simulink model "gm_CustArch"  (R2020a)
settings: Solver=FixedStepDiscrete  StartTime=0.0  StopTime=7e4  RelTol=1e-3
libraries: simulink x85, hdlsllib x52, hdlmdlgenlib x2
(part 1 of 3)
settings Model: FPTRunName=FPA_Reference  Creator=BuccelliLab  LastModifiedBy=diflo
settings SolverCC: AutoInsertRateTranBlk=on  MinimalZcImpactIntegration=on
settings DataIOCC: LimitDataPoints=on  SaveOutput=off  SaveTime=off  ReturnWorkspaceOutputs=off
settings OptimizationCC: BlockReduction=off  ConditionallyExecuteInputs=off  DefaultParameterBehavior=Inlined  LifeSpan=inf
settings DebuggingCC: SignalRangeChecking=warning  ReadBeforeWriteMsg=DisableAll  WriteAfterWriteMsg=DisableAll  WriteAfterReadMsg=DisableAll  AlgebraicLoopMsg=error  ArtificialAlgebraicLoopMsg=none  InheritedTsInSrcMsg=none  MultiTaskDSMMsg=none  SingleTaskRateTransMsg=error  ParameterDowncastMsg=warning  ParameterOverflowMsg=warning  AllowSymbolicDim=off  StrictBusMsg=ErrorOnBusTreatedAsVector  SFUnexpectedBacktrackingDiag=warning  SFNoUnconditionalDefaultTransitionDiag=warning  SFExecutionAtInitializationDiag=none  ArithmeticOperatorsInVariantConditions=warning
settings HardwareCC: ProdBitPerPointer=32  ProdBitPerSizeT=32  ProdBitPerPtrDiffT=32  ProdLargestAtomicFloat=None  ProdIntDivRoundTo=Undefined  ProdEndianess=Unspecified  ProdWordSize=32  ProdHWDeviceType=ASIC/FPGA->ASIC/FPGA  TargetBitPerPointer=64  TargetBitPerSizeT=64  TargetBitPerPtrDiffT=64  TargetLongLongMode=on  TargetIntDivRoundTo=Zero  TargetEndianess=LittleEndian  TargetWordSize=64  TargetHWDeviceType=Custom Processor->MATLAB Host Computer  ProdEqTarget=off
settings ModelReferenceCC: UpdateModelReferenceTargets=IfOutOfDate
settings SFSimCC: SFSimEcho=off  SimUseLocalCustomCode=off  CustomCodeUndefinedFunction=UseInterfaceOnly
settings RTWCC: RTWUseLocalCustomCode=off
settings CodeAppCC: StateflowObjectComments=on
settings GRTTargetCC: TargetLangStandard=C89/C90 (ANSI)
settings ConfigComp: CovScope=ReferencedModels  CovMetricSettings=dw  CovHtmlReporting=on  CovSaveCumulativeToWorkspaceVar=on  CovSaveSingleToWorkspaceVar=on  CovExternalEMLEnable=off  CovSFcnEnable=off

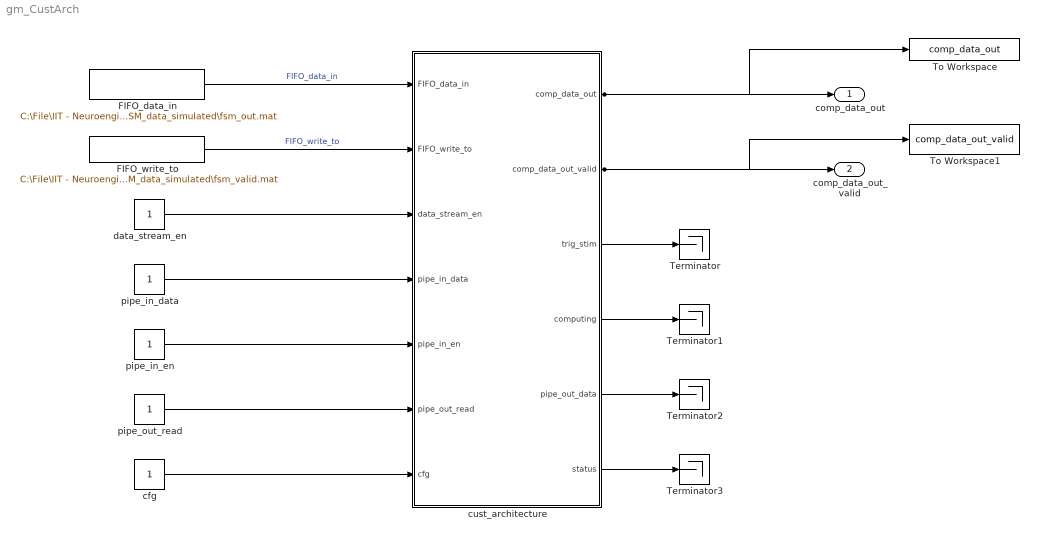
== system gm_CustArch ==
  FIFO_data_in : FromFile  FileName=C:\File\IIT - Neuroengineering\Progetto MathWorks\Data\Intan recordings\FSM_data_simulated\fsm_out.mat  OutDataTypeStr=uint16  SampleTime=1  ExtrapolationBeforeFirstDataPoint=Hold first value  InterpolationWithinTimeRange=Zero order hold  ExtrapolationAfterLastDataPoint=Hold last value
  FIFO_write_to : FromFile  FileName=C:\File\IIT - Neuroengineering\Progetto MathWorks\Data\Intan recordings\FSM_data_simulated\fsm_valid.mat  OutDataTypeStr=boolean  SampleTime=1
  Terminator{,1..3} (4 alike) : Terminator
  To Workspace : ToWorkspace  VariableName=comp_data_out  SaveFormat=Timeseries  SampleTime=-1
  To Workspace1 : ToWorkspace  VariableName=comp_data_out_valid  SaveFormat=Timeseries  SampleTime=-1
  cfg : Constant  OutDataTypeStr=uint16  SampleTime=-1
  cust_architecture : Subsystem
  data_stream_en : Constant  OutDataTypeStr=uint8  SampleTime=-1
  pipe_in_data : Constant  OutDataTypeStr=uint16  SampleTime=-1
  pipe_in_en : Constant  OutDataTypeStr=boolean  SampleTime=-1
  pipe_out_read : Constant  OutDataTypeStr=boolean  SampleTime=-1
  comp_data_out : Outport  VectorParamsAs1DForOutWhenUnconnected=off
  comp_data_out_valid : Outport  Port=2  VectorParamsAs1DForOutWhenUnconnected=off
  wires:
  cust_architecture/6(status) -> Terminator3/1
  cust_architecture/5(pipe_out_data) -> Terminator2/1
  cust_architecture/4(computing) -> Terminator1/1
  cust_architecture/3(trig_stim) -> Terminator/1
  cfg/1 -> cust_architecture/7(cfg)
  pipe_out_read/1 -> cust_architecture/6(pipe_out_read)
  pipe_in_en/1 -> cust_architecture/5(pipe_in_en)
  pipe_in_data/1 -> cust_architecture/4(pipe_in_data)
  data_stream_en/1 -> cust_architecture/3(data_stream_en)
  cust_architecture/2(comp_data_out_valid) -> comp_data_out_valid/1, To Workspace1/1
  cust_architecture/1(comp_data_out) -> comp_data_out/1, To Workspace/1
  FIFO_write_to/1 -> cust_architecture/2(FIFO_write_to)  "FIFO_write_to"
  FIFO_data_in/1 -> cust_architecture/1(FIFO_data_in)  "FIFO_data_in"

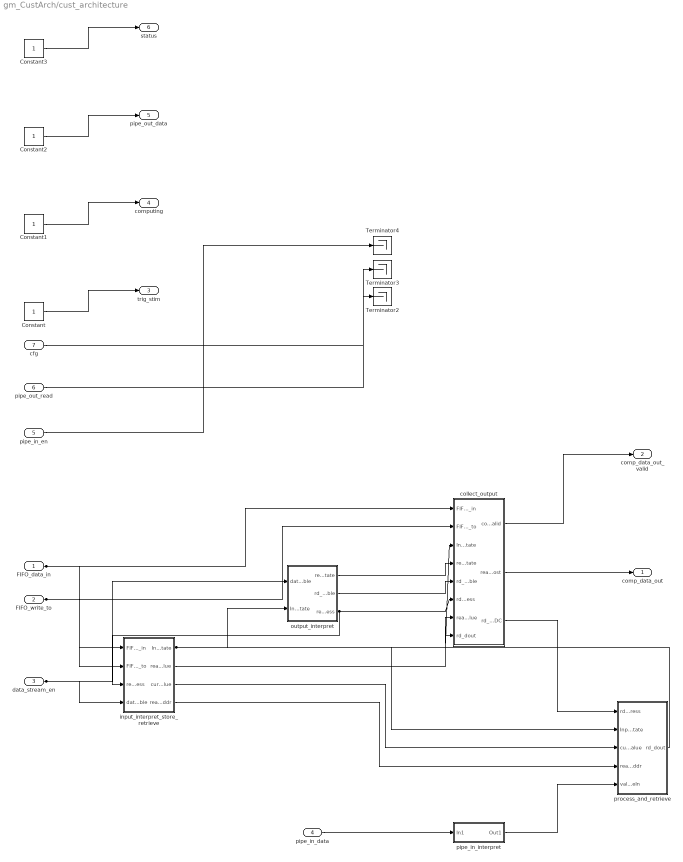
== system gm_CustArch/cust_architecture ==
  FIFO_data_in : Inport  OutDataTypeStr=uint16  PortDimensions=1  SampleTime=1
  FIFO_write_to : Inport  Port=2  OutDataTypeStr=boolean  PortDimensions=1  SampleTime=1
  data_stream_en : Inport  Port=3  OutDataTypeStr=uint8  PortDimensions=1  SampleTime=1
  pipe_in_data : Inport  Port=4  OutDataTypeStr=uint16  PortDimensions=1  SampleTime=1
  pipe_in_en : Inport  Port=5  OutDataTypeStr=boolean  PortDimensions=1  SampleTime=1
  pipe_out_read : Inport  Port=6  OutDataTypeStr=boolean  PortDimensions=1  SampleTime=1
  cfg : Inport  Port=7  OutDataTypeStr=uint16  PortDimensions=1  SampleTime=1
  Constant : Constant  OutDataTypeStr=uint8  SampleTime=1
  Constant1 : Constant  OutDataTypeStr=boolean  SampleTime=1
  Constant2 : Constant  OutDataTypeStr=uint16  SampleTime=1
  Constant3 : Constant  OutDataTypeStr=uint16  SampleTime=1
  Terminator2 : Terminator
  Terminator3 : Terminator
  Terminator4 : Terminator
  collect_output : Subsystem
  input_interpret_store_retrieve : Subsystem
  output_interpret : Subsystem
  pipe_in_interpret : Subsystem
  process_and_retrieve : Subsystem
  comp_data_out : Outport  VectorParamsAs1DForOutWhenUnconnected=off
  comp_data_out_valid : Outport  Port=2  OutDataTypeStr=boolean  VectorParamsAs1DForOutWhenUnconnected=off
  trig_stim : Outport  Port=3  VectorParamsAs1DForOutWhenUnconnected=off
  computing : Outport  Port=4  VectorParamsAs1DForOutWhenUnconnected=off
  pipe_out_data : Outport  Port=5  VectorParamsAs1DForOutWhenUnconnected=off
  status : Outport  Port=6  VectorParamsAs1DForOutWhenUnconnected=off
  wires:
  FIFO_data_in/1 -> input_interpret_store_retrieve/1(FIFO_data_in), collect_output/1(FIFO_data_in)
  FIFO_write_to/1 -> collect_output/2(FIFO_write_to), input_interpret_store_retrieve/2(FIFO_write_to)
  data_stream_en/1 -> output_interpret/1(data_stream_enable), input_interpret_store_retrieve/4(data_stream_enable)
  pipe_in_data/1 -> pipe_in_interpret/1(In1)
  pipe_in_en/1 -> Terminator4/1
  pipe_out_read/1 -> Terminator3/1
  cfg/1 -> Terminator2/1
  Constant/1 -> trig_stim/1
  Constant1/1 -> computing/1
  Constant2/1 -> pipe_out_data/1
  Constant3/1 -> status/1
  collect_output/1(comp_data_out_valid) -> comp_data_out_valid/1
  collect_output/2(read_from_storage_post) -> comp_data_out/1
  collect_output/3(rd_address_bit_set_AC_during_DC) -> process_and_retrieve/1(rd_address)
  input_interpret_store_retrieve/1(InputState) -> collect_output/3(InputState), output_interpret/2(InputState), process_and_retrieve/2(InputState)
  input_interpret_store_retrieve/2(read_from_storage_value) -> collect_output/7(read_from_storage_value)
  input_interpret_store_retrieve/3(current_value) -> process_and_retrieve/3(current_value)
  input_interpret_store_retrieve/4(read_from_processing_addr) -> process_and_retrieve/4(read_from_processing_addr)
  output_interpret/1(read_address == output_state) -> collect_output/4(read_address == output_state)
  output_interpret/2(rd_enable) -> collect_output/5(rd_enable)
  output_interpret/3(read_address) -> collect_output/6(rd_address), input_interpret_store_retrieve/3(read_address)
  pipe_in_interpret/1(Out1) -> process_and_retrieve/5(value_from_pipeIn)
  process_and_retrieve/1(rd_dout) -> collect_output/8(rd_dout)

== system gm_CustArch/cust_architecture/collect_output ==
  FIFO_data_in : Inport  OutDataTypeStr=uint16  PortDimensions=1  SampleTime=1
  FIFO_write_to : Inport  Port=2  OutDataTypeStr=boolean  PortDimensions=1  SampleTime=1
  InputState : Inport  Port=3  OutDataTypeStr=uint8  PortDimensions=1  SampleTime=1
  read_address == output_state : Inport  Port=4  OutDataTypeStr=uint8  PortDimensions=1  SampleTime=1
  rd_enable : Inport  Port=5  OutDataTypeStr=boolean  PortDimensions=1  SampleTime=1
  rd_address : Inport  Port=6  OutDataTypeStr=fixdt(0, 9, 0)  PortDimensions=1  SampleTime=1
  read_from_storage_value : Inport  Port=7  OutDataTypeStr=uint16  PortDimensions=1  SampleTime=1
  rd_dout : Inport  Port=8  OutDataTypeStr=uint16  PortDimensions=1  SampleTime=1
  AND : Logic  AllPortsSameDT=off  OutDataTypeStr=boolean  SampleTime=1
  Bit Set to get AC during DC : simulink/Logic and Bit Operations/Bit Set  iBit=0
      settings: SourceProductBaseCode=SL
  Compare To Constant : simulink/Logic and Bit Operations/Compare To Constant  relop=<  const="fi(0,0,8,0,\"hex\",\"06\")"  OutDataTypeStr=boolean
  Memory : UnitDelay  InitialCondition=double(0)  SampleTime=1
  Memory1 : UnitDelay  InitialCondition=double(0)  SampleTime=1
  Memory7 : UnitDelay  InitialCondition=double(0)  SampleTime=1
  Switch : Switch  Criteria=u2 > Threshold  Threshold=double(0)  OutDataTypeStr=uint16  SampleTime=1
  Switch2 : Switch  Criteria=u2 > Threshold  Threshold=double(0)  OutDataTypeStr=uint16  SampleTime=1
  get_data only when enabled : Subsystem
  output_state_DC : simulink/Logic and Bit Operations/Compare To Constant  relop=~=  const="fi(0,0,8,0,\"hex\",\"06\")"  OutDataTypeStr=boolean
  read_from_magic_and_timestamp : Subsystem
  comp_data_out_valid : Outport
  read_from_storage_post : Outport  Port=2
  rd_address_bit_set_AC_during_DC : Outport  Port=3
  wires:
  FIFO_data_in/1 -> read_from_magic_and_timestamp/2(FIFO_data_in)
  FIFO_write_to/1 -> read_from_magic_and_timestamp/3(FIFO_write_to)
  InputState/1 -> read_from_magic_and_timestamp/4(InputState)
  read_address == output_state/1 -> output_state_DC/1, Memory/1, read_from_magic_and_timestamp/1(read_address == output_state)
  rd_enable/1 -> Memory1/1
  rd_address/1 -> Bit Set to get AC during DC/1
  read_from_storage_value/1 -> Switch2/1
  rd_dout/1 -> Switch2/3
  AND/1 -> Switch/2
  Bit Set to get AC during DC/1 -> rd_address_bit_set_AC_during_DC/1
  Compare To Constant/1 -> AND/1
  Memory/1 -> Compare To Constant/1
  Memory1/1 -> AND/2, comp_data_out_valid/1, get_data only when enabled/Enable
  Memory7/1 -> Switch2/2
  Switch/1 -> get_data only when enabled/1(In1)
  Switch2/1 -> Switch/3
  get_data only when enabled/1(Out1) -> read_from_storage_post/1
  output_state_DC/1 -> Memory7/1
  read_from_magic_and_timestamp/1(read_from_Magic_TS) -> Switch/1

== system gm_CustArch/cust_architecture/input_interpret_store_retrieve ==
  FIFO_data_in : Inport  OutDataTypeStr=uint16  PortDimensions=1  SampleTime=1
  FIFO_write_to : Inport  Port=2  OutDataTypeStr=boolean  PortDimensions=1  SampleTime=1
  read_address : Inport  Port=3  OutDataTypeStr=fixdt(0, 9, 0)  PortDimensions=1  SampleTime=1
  data_stream_enable : Inport  Port=4  OutDataTypeStr=uint8  PortDimensions=1  SampleTime=1
  InputStateMachine : Subsystem
  Interpret_to_RAM_input : Subsystem
  store_and_retrieve_input : Subsystem
  InputState : Outport
  read_from_storage_value : Outport  Port=2
  current_value : Outport  Port=3
  read_from_processing_addr : Outport  Port=4
  wires:
  FIFO_data_in/1 -> InputStateMachine/1(FIFO_data_in), Interpret_to_RAM_input/1(FIFO_data_in)
  FIFO_write_to/1 -> InputStateMachine/2(FIFO_write_to), Interpret_to_RAM_input/2(FIFO_write_to)
  read_address/1 -> store_and_retrieve_input/1(read address)
  data_stream_enable/1 -> Interpret_to_RAM_input/4(data_stream_enable)
  InputStateMachine/1(InputState) -> InputState/1, Interpret_to_RAM_input/3(InputState)
  Interpret_to_RAM_input/1(device_output) -> InputStateMachine/3(channel_0_19)
  Interpret_to_RAM_input/2(inc_source_device) -> InputStateMachine/4(inc_source_device_MSB)
  Interpret_to_RAM_input/3(wr_din) -> store_and_retrieve_input/2(wr_din)
  Interpret_to_RAM_input/4(write address) -> store_and_retrieve_input/3(wr_address)
  Interpret_to_RAM_input/5(wr_en) -> store_and_retrieve_input/4(wr_en)
  store_and_retrieve_input/1(read_from_storage_value) -> read_from_storage_value/1
  store_and_retrieve_input/2(current value) -> current_value/1
  store_and_retrieve_input/3(read_from_porcessing_addr) -> read_from_processing_addr/1

== system gm_CustArch/cust_architecture/output_interpret ==
  data_stream_enable : Inport  OutDataTypeStr=uint8  PortDimensions=1  SampleTime=1
  InputState : Inport  Port=2  OutDataTypeStr=uint8  PortDimensions=1  SampleTime=1
  Interpret_to_RAM_output : Subsystem
  OutputStateMachine : Subsystem
  read_address == output_state : Outport
  rd_enable : Outport  Port=2
  read_address : Outport  Port=3
  wires:
  data_stream_enable/1 -> Interpret_to_RAM_output/2(data_stream_en)
  InputState/1 -> OutputStateMachine/1(input_state)
  Interpret_to_RAM_output/1(rd_enable) -> rd_enable/1
  Interpret_to_RAM_output/2(read address) -> read_address/1
  OutputStateMachine/1(OutputState) -> read_address == output_state/1, Interpret_to_RAM_output/1(read_address == output_state)

== system gm_CustArch/cust_architecture/pipe_in_interpret ==
  In1 : Inport  OutDataTypeStr=uint16  PortDimensions=1  SampleTime=1
  Bit Slice1 : hdlsllib/Logic and Bit Operations/Bit Slice  lidx=double(15)  ridx=double(8)
      settings: SourceProductBaseCode=SL
  Compare To Constant1 : simulink/Logic and Bit Operations/Compare To Constant  relop===  const="fi(0,0,8,0,\"hex\",\"02\")"  OutDataTypeStr=boolean
  Constant4 : Constant  Value=5  OutDataTypeStr=uint16  SampleTime=1
  Memory6 : UnitDelay  InitialCondition=double(0)  SampleTime=1
  Switch1 : Switch  Criteria=u2 > Threshold  Threshold=double(0)  OutDataTypeStr=uint16  SampleTime=1
  Out1 : Outport
  wires:
  In1/1 -> Switch1/1, Memory6/1
  Bit Slice1/1 -> Compare To Constant1/1
  Compare To Constant1/1 -> Switch1/2
  Constant4/1 -> Switch1/3
  Memory6/1 -> Bit Slice1/1
  Switch1/1 -> Out1/1

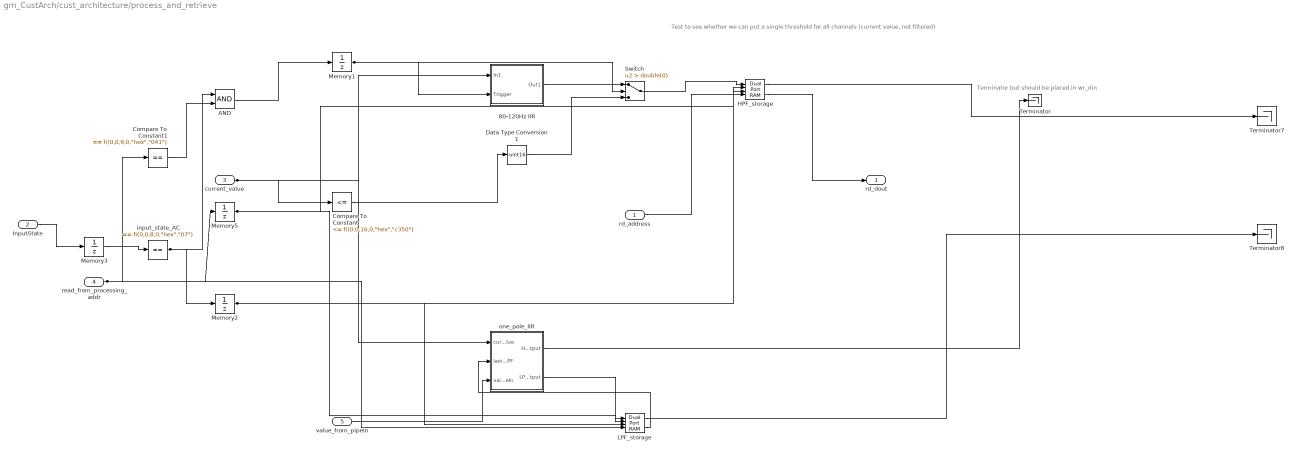
== system gm_CustArch/cust_architecture/process_and_retrieve ==
  note: Terminator but should be placed in wr_din
  note: Test to see whether we can put a single threshold for all channels (current value, not filtered)
  rd_address : Inport  OutDataTypeStr=fixdt(0, 9, 0)  PortDimensions=1  SampleTime=1
  InputState : Inport  Port=2  OutDataTypeStr=uint8  PortDimensions=1  SampleTime=1
  current_value : Inport  Port=3  OutDataTypeStr=uint16  PortDimensions=1  SampleTime=1
  read_from_processing_addr : Inport  Port=4  OutDataTypeStr=fixdt(0, 9, 0)  PortDimensions=1  SampleTime=1
  value_from_pipeIn : Inport  Port=5  OutDataTypeStr=uint16  PortDimensions=1  SampleTime=1
  80-120Hz IIR : Subsystem
  AND : Logic  AllPortsSameDT=off  OutDataTypeStr=boolean  SampleTime=1
  Compare To Constant : simulink/Logic and Bit Operations/Compare To Constant  relop=<=  const="fi(0,0,16,0,\"hex\",\"c350\")"  OutDataTypeStr=boolean
  Compare To Constant1 : simulink/Logic and Bit Operations/Compare To Constant  relop===  const="fi(0,0,9,0,\"hex\",\"041\")"  OutDataTypeStr=boolean
  Data Type Conversion1 : DataTypeConversion  OutDataTypeStr=uint16  SampleTime=1  SaturateOnIntegerOverflow=on
  HPF_storage : hdlsllib/HDL RAMs/Dual Port RAM  ram_size=9
      settings: SourceProductBaseCode=SL
  LPF_storage : hdlsllib/HDL RAMs/Dual Port RAM  ram_size=9
      settings: SourceProductBaseCode=SL
  Memory{1..3,5} (4 alike) : UnitDelay  InitialCondition=double(0)  SampleTime=1
  Switch : Switch  Criteria=u2 > Threshold  Threshold=double(0)  OutDataTypeStr=uint16  SampleTime=1
  Terminator : Terminator
  Terminator7 : Terminator
  Terminator8 : Terminator
  input_state_AC : simulink/Logic and Bit Operations/Compare To Constant  relop===  const="fi(0,0,8,0,\"hex\",\"07\")"  OutDataTypeStr=boolean
  one_pole_IIR : Subsystem
  rd_dout : Outport
  wires:
  rd_address/1 -> HPF_storage/4
  InputState/1 -> Memory3/1
  current_value/1 -> Compare To Constant/1, one_pole_IIR/1(current_value), 80-120Hz IIR/1(In1)
  read_from_processing_addr/1 -> Compare To Constant1/1, Memory5/1, LPF_storage/4
  value_from_pipeIn/1 -> one_pole_IIR/3(value_from_pipeIn)
  80-120Hz IIR/1(Out1) -> Switch/1
  AND/1 -> Memory1/1
  Compare To Constant/1 -> Data Type Conversion1/1
  Compare To Constant1/1 -> AND/2
  Data Type Conversion1/1 -> Switch/3
  HPF_storage/1 -> Terminator7/1
  HPF_storage/2 -> rd_dout/1
  LPF_storage/1 -> Terminator8/1
  LPF_storage/2 -> one_pole_IIR/2(last_LPF)
  Memory1/1 -> Switch/2, 80-120Hz IIR/2(Trigger)
  Memory2/1 -> HPF_storage/3, LPF_storage/3
  Memory3/1 -> input_state_AC/1
  Memory5/1 -> HPF_storage/2, LPF_storage/2
  Switch/1 -> HPF_storage/1
  input_state_AC/1 -> AND/1, Memory2/1
  one_pole_IIR/1(HPF_output) -> Terminator/1
  one_pole_IIR/2(LPF_output) -> LPF_storage/1

== system gm_CustArch/cust_architecture/collect_output/get_data only when enabled ==
  In1 : Inport  OutDataTypeStr=uint16  PortDimensions=1  SampleTime=1
  Enable : EnablePort  OutDataTypeStr=boolean
  Out1 : Outport  InitialOutput=0  VectorParamsAs1DForOutWhenUnconnected=off
  wires:
  In1/1 -> Out1/1

== system gm_CustArch/cust_architecture/collect_output/read_from_magic_and_timestamp ==
  read_address == output_state : Inport  OutDataTypeStr=uint8  PortDimensions=1  SampleTime=1
  FIFO_data_in : Inport  Port=2  OutDataTypeStr=uint16  PortDimensions=1  SampleTime=1
  FIFO_write_to : Inport  Port=3  OutDataTypeStr=boolean  PortDimensions=1  SampleTime=1
  InputState : Inport  Port=4  OutDataTypeStr=uint8  PortDimensions=1  SampleTime=1
  Terminator1 : Terminator
  getting address and enable for Magic and Timestamps : Subsystem
  input_RAM_for_MagicNumber_TimeStamps : hdlsllib/HDL RAMs/Dual Port RAM  ram_size=8
      settings: SourceProductBaseCode=SL
  read_from_Magic_TS : Outport
  wires:
  read_address == output_state/1 -> input_RAM_for_MagicNumber_TimeStamps/4
  FIFO_data_in/1 -> input_RAM_for_MagicNumber_TimeStamps/1
  FIFO_write_to/1 -> getting address and enable for Magic and Timestamps/2(FIFO_write_to)
  InputState/1 -> getting address and enable for Magic and Timestamps/1(InputState)
  getting address and enable for Magic and Timestamps/1(wr_address) -> input_RAM_for_MagicNumber_TimeStamps/2
  getting address and enable for Magic and Timestamps/2(wr_enable) -> input_RAM_for_MagicNumber_TimeStamps/3
  input_RAM_for_MagicNumber_TimeStamps/1 -> Terminator1/1
  input_RAM_for_MagicNumber_TimeStamps/2 -> read_from_Magic_TS/1

== system gm_CustArch/cust_architecture/input_interpret_store_retrieve/InputStateMachine ==
  FIFO_data_in : Inport  OutDataTypeStr=uint16  PortDimensions=1  SampleTime=1
  FIFO_write_to : Inport  Port=2  OutDataTypeStr=boolean  PortDimensions=1  SampleTime=1
  channel_0_19 : Inport  Port=3  OutDataTypeStr=uint8  PortDimensions=1  SampleTime=1
  inc_source_device_MSB : Inport  Port=4  OutDataTypeStr=boolean  PortDimensions=1  SampleTime=1
  InputStateMachine : Stateflow chart  TreatAsAtomicUnit=on
  InputState : Outport  VectorParamsAs1DForOutWhenUnconnected=off
  wires:
  FIFO_data_in/1 -> InputStateMachine/1(FIFO_data_in)
  FIFO_write_to/1 -> InputStateMachine/2(FIFO_write_to)
  channel_0_19/1 -> InputStateMachine/3(channel_0_19)
  inc_source_device_MSB/1 -> InputStateMachine/4(inc_source_device_MSB)
  InputStateMachine/1(InputState) -> InputState/1

== system gm_CustArch/cust_architecture/input_interpret_store_retrieve/Interpret_to_RAM_input ==
  FIFO_data_in : Inport  OutDataTypeStr=uint16  PortDimensions=1  SampleTime=1
  FIFO_write_to : Inport  Port=2  OutDataTypeStr=boolean  PortDimensions=1  SampleTime=1
  InputState : Inport  Port=3  OutDataTypeStr=uint8  PortDimensions=1  SampleTime=1
  data_stream_enable : Inport  Port=4  OutDataTypeStr=uint8  PortDimensions=1  SampleTime=1
  Input State to RAM address (to write) : Subsystem
  interpret data : Subsystem
  device_output : Outport
  inc_source_device : Outport  Port=2
  wr_din : Outport  Port=3
  write address : Outport  Port=4
  wr_en : Outport  Port=5
  wires:
  FIFO_data_in/1 -> Input State to RAM address (to write)/1(DataIn)
  FIFO_write_to/1 -> Input State to RAM address (to write)/6(write_to), interpret data/1(FIFO_write_to)
  InputState/1 -> Input State to RAM address (to write)/2(InputState), interpret data/2(InputState)
  data_stream_enable/1 -> interpret data/3(data_stream_enable)
  Input State to RAM address (to write)/1(wr_din) -> wr_din/1
  Input State to RAM address (to write)/2(wr_addr) -> write address/1
  Input State to RAM address (to write)/3(write_enable_6to15) -> wr_en/1
  interpret data/1(source_device) -> Input State to RAM address (to write)/4(source_device)
  interpret data/2(inc_source_device) -> inc_source_device/1
  interpret data/3(device_output) -> device_output/1
  interpret data/4(source_channel_0_159) -> Input State to RAM address (to write)/3(source_channel_0_159)
  interpret data/5(converter_cnt) -> Input State to RAM address (to write)/5(converter_cnt)

== system gm_CustArch/cust_architecture/input_interpret_store_retrieve/store_and_retrieve_input ==
  note: salvataggio dati su dual-ram, ogni dato ha un indirizzo associato
  note: così so l'indirizzo del dato
  read address : Inport  OutDataTypeStr=fixdt(0, 9, 0)  PortDimensions=1  SampleTime=1
  wr_din : Inport  Port=2  OutDataTypeStr=uint16  PortDimensions=1  SampleTime=1
  wr_address : Inport  Port=3  OutDataTypeStr=fixdt(0, 9, 0)  PortDimensions=1  SampleTime=1
  wr_en : Inport  Port=4  OutDataTypeStr=boolean  PortDimensions=1  SampleTime=1
  Memory4 : UnitDelay  InitialCondition=double(0)  SampleTime=1
  Terminator : Terminator
  Terminator6 : Terminator
  input_storage : hdlsllib/HDL RAMs/Dual Port RAM  ram_size=9
      settings: SourceProductBaseCode=SL
  input_storage_for_processing : hdlsllib/HDL RAMs/Dual Port RAM  ram_size=9
      settings: SourceProductBaseCode=SL
  read_from_storage_value : Outport
  current value : Outport  Port=2
  read_from_porcessing_addr : Outport  Port=3
  wires:
  read address/1 -> input_storage/4
  wr_din/1 -> input_storage/1, input_storage_for_processing/1
  wr_address/1 -> Memory4/1, input_storage/2, input_storage_for_processing/2
  wr_en/1 -> input_storage/3, input_storage_for_processing/3
  Memory4/1 -> read_from_porcessing_addr/1, input_storage_for_processing/4
  input_storage/1 -> Terminator/1
  input_storage/2 -> read_from_storage_value/1
  input_storage_for_processing/1 -> Terminator6/1
  input_storage_for_processing/2 -> current value/1

== system gm_CustArch/cust_architecture/output_interpret/Interpret_to_RAM_output ==
  read_address == output_state : Inport  OutDataTypeStr=uint8  PortDimensions=1  SampleTime=1
  data_stream_en : Inport  Port=2  OutDataTypeStr=uint8  PortDimensions=1  SampleTime=1
  Output State to RAM address (to read) : Subsystem
  "get enabled timings " : Subsystem
  rd_enable : Outport
  read address : Outport  Port=2
  wires:
  read_address == output_state/1 -> Output State to RAM address (to read)/3(OutputState), "get enabled timings "/1(output_state)
  data_stream_en/1 -> "get enabled timings "/2(data_stream_en)
  Output State to RAM address (to read)/1(rd_enable) -> rd_enable/1
  Output State to RAM address (to read)/2(rd_addr) -> read address/1
  "get enabled timings "/1(source_channel_en) -> Output State to RAM address (to read)/1(source_channel_en)
  "get enabled timings "/2(source_ch_0_159) -> Output State to RAM address (to read)/2(source_channel)
  "get enabled timings "/3(source_device_enabled) -> Output State to RAM address (to read)/4(source_device_en)
  "get enabled timings "/4(source_device) -> Output State to RAM address (to read)/5(source_device)
  "get enabled timings "/5(converter_cnt) -> Output State to RAM address (to read)/6(converter_cnt)

== system gm_CustArch/cust_architecture/output_interpret/OutputStateMachine ==
  input_state : Inport  OutDataTypeStr=uint8  PortDimensions=1  SampleTime=1
  OutputStateMachine : Stateflow chart  TreatAsAtomicUnit=on
  OutputState : Outport  VectorParamsAs1DForOutWhenUnconnected=off
  wires:
  input_state/1 -> OutputStateMachine/1(input_state)
  OutputStateMachine/1(OutputState) -> OutputState/1

== system gm_CustArch/cust_architecture/process_and_retrieve/80-120Hz IIR ==
  In1 : Inport  OutDataTypeStr=uint16  PortDimensions=1  SampleTime=1
  Trigger : Inport  Port=2  OutDataTypeStr=boolean  SampleTime=1
  Trigger_delay : Delay  DelayLength=double(1)  InitialCondition=1
  Trigger_delayed_inverted_and_Trigger : Logic  AllPortsSameDT=off  OutDataTypeStr=boolean  SampleTime=1
  controlss_temp : Subsystem
  not_Trigger_delayed : Logic  Operator=NOT  Inputs=1  AllPortsSameDT=off  OutDataTypeStr=boolean  SampleTime=1
  Out1 : Outport  InitialOutput=0
  wires:
  Trigger/1 -> Trigger_delayed_inverted_and_Trigger/2, Trigger_delay/1
  In1/1 -> controlss_temp/1(in0)
  controlss_temp/1(out0) -> Out1/1
  Trigger_delay/1 -> not_Trigger_delayed/1
  not_Trigger_delayed/1 -> Trigger_delayed_inverted_and_Trigger/1
  Trigger_delayed_inverted_and_Trigger/1 -> controlss_temp/2(Trigger_emulated)

== system gm_CustArch/cust_architecture/process_and_retrieve/one_pole_IIR ==
  current_value : Inport  OutDataTypeStr=uint16  PortDimensions=1  SampleTime=1
  last_LPF : Inport  Port=2  OutDataTypeStr=fixdt(1, 16, -5)  PortDimensions=1  SampleTime=1
  value_from_pipeIn : Inport  Port=3  OutDataTypeStr=uint16  PortDimensions=1  SampleTime=1
  Constant : Constant  Value=32768  OutDataTypeStr=uint16  SampleTime=1
  Constant1 : Constant  Value=32768  OutDataTypeStr=uint16  SampleTime=1
  Data Type Conversion1 : DataTypeConversion  OutDataTypeStr=int16  SampleTime=1  SaturateOnIntegerOverflow=on
  Filter1 : Subsystem
  Subtract1 : Sum  Inputs=+-  AccumDataTypeStr=fixdt(1, 17, 0)  OutDataTypeStr=int16  SampleTime=1
  Subtract2 : Sum  AccumDataTypeStr=fixdt(1, 18, 0)  OutDataTypeStr=uint16  SampleTime=1
  Terminator : Terminator
  HPF_output : Outport  VectorParamsAs1DForOutWhenUnconnected=off
  LPF_output : Outport  Port=2  VectorParamsAs1DForOutWhenUnconnected=off
  wires:
  current_value/1 -> Subtract1/1
  last_LPF/1 -> Filter1/2(Input1)
  value_from_pipeIn/1 -> Terminator/1
  Constant/1 -> Subtract1/2
  Constant1/1 -> Subtract2/2
  Data Type Conversion1/1 -> Subtract2/1
  Filter1/1(Output) -> Data Type Conversion1/1
  Filter1/2(Output1) -> LPF_output/1
  Subtract1/1 -> Filter1/1(Input)
  Subtract2/1 -> HPF_output/1

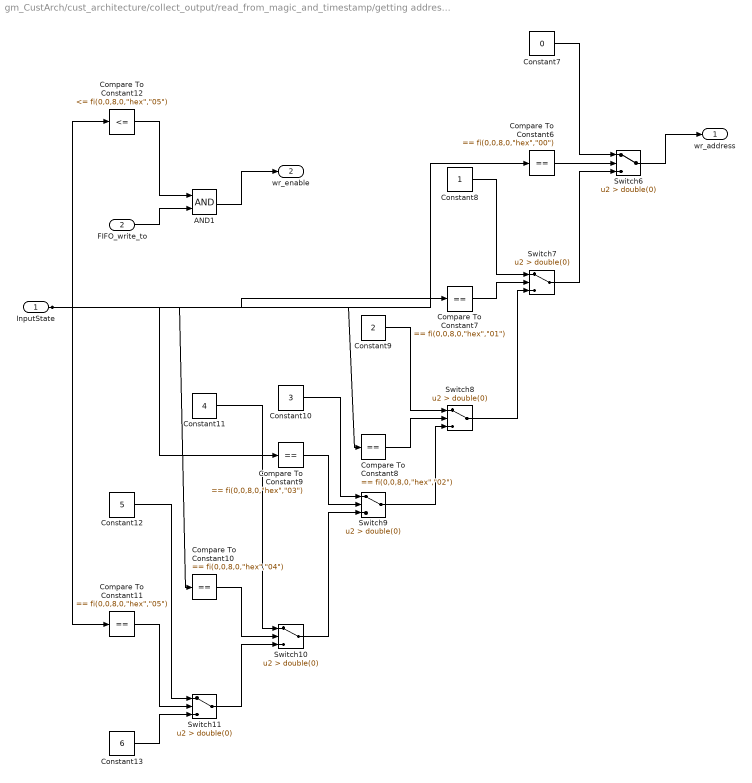
== system gm_CustArch/cust_architecture/collect_output/read_from_magic_and_timestamp/getting address and enable for Magic and Timestamps ==
  InputState : Inport  OutDataTypeStr=uint8  PortDimensions=1  SampleTime=1
  FIFO_write_to : Inport  Port=2  OutDataTypeStr=boolean  PortDimensions=1  SampleTime=1
  AND1 : Logic  AllPortsSameDT=off  OutDataTypeStr=boolean  SampleTime=1
  Compare To Constant10 : simulink/Logic and Bit Operations/Compare To Constant  relop===  const="fi(0,0,8,0,\"hex\",\"04\")"  OutDataTypeStr=boolean
  Compare To Constant11 : simulink/Logic and Bit Operations/Compare To Constant  relop===  const="fi(0,0,8,0,\"hex\",\"05\")"  OutDataTypeStr=boolean
  Compare To Constant12 : simulink/Logic and Bit Operations/Compare To Constant  relop=<=  const="fi(0,0,8,0,\"hex\",\"05\")"  OutDataTypeStr=boolean
  Compare To Constant6 : simulink/Logic and Bit Operations/Compare To Constant  relop===  const="fi(0,0,8,0,\"hex\",\"00\")"  OutDataTypeStr=boolean
  Compare To Constant7 : simulink/Logic and Bit Operations/Compare To Constant  relop===  const="fi(0,0,8,0,\"hex\",\"01\")"  OutDataTypeStr=boolean
  Compare To Constant8 : simulink/Logic and Bit Operations/Compare To Constant  relop===  const="fi(0,0,8,0,\"hex\",\"02\")"  OutDataTypeStr=boolean
  Compare To Constant9 : simulink/Logic and Bit Operations/Compare To Constant  relop===  const="fi(0,0,8,0,\"hex\",\"03\")"  OutDataTypeStr=boolean
  Constant10 : Constant  Value=3  OutDataTypeStr=uint8  SampleTime=1
  Constant11 : Constant  Value=4  OutDataTypeStr=uint8  SampleTime=1
  Constant12 : Constant  Value=5  OutDataTypeStr=uint8  SampleTime=1
  Constant13 : Constant  Value=6  OutDataTypeStr=uint8  SampleTime=1
  Constant7 : Constant  Value=0  OutDataTypeStr=uint8  SampleTime=1
  Constant8 : Constant  OutDataTypeStr=uint8  SampleTime=1
  Constant9 : Constant  Value=2  OutDataTypeStr=uint8  SampleTime=1
  Switch{6..11} (6 alike) : Switch  Criteria=u2 > Threshold  Threshold=double(0)  OutDataTypeStr=uint8  SampleTime=1
  wr_address : Outport  VectorParamsAs1DForOutWhenUnconnected=off
  wr_enable : Outport  Port=2  VectorParamsAs1DForOutWhenUnconnected=off
  wires:
  InputState/1 -> Compare To Constant9/1, Compare To Constant8/1, Compare To Constant7/1, Compare To Constant6/1, Compare To Constant12/1, Compare To Constant11/1, Compare To Constant10/1
  FIFO_write_to/1 -> AND1/2
  AND1/1 -> wr_enable/1
  Compare To Constant10/1 -> Switch10/2
  Compare To Constant11/1 -> Switch11/2
  Compare To Constant12/1 -> AND1/1
  Compare To Constant6/1 -> Switch6/2
  Compare To Constant7/1 -> Switch7/2
  Compare To Constant8/1 -> Switch8/2
  Compare To Constant9/1 -> Switch9/2
  Constant10/1 -> Switch9/1
  Constant11/1 -> Switch10/1
  Constant12/1 -> Switch11/1
  Constant13/1 -> Switch11/3
  Constant7/1 -> Switch6/1
  Constant8/1 -> Switch7/1
  Constant9/1 -> Switch8/1
  Switch10/1 -> Switch9/3
  Switch11/1 -> Switch10/3
  Switch6/1 -> wr_address/1
  Switch7/1 -> Switch6/3
  Switch8/1 -> Switch7/3
  Switch9/1 -> Switch8/3

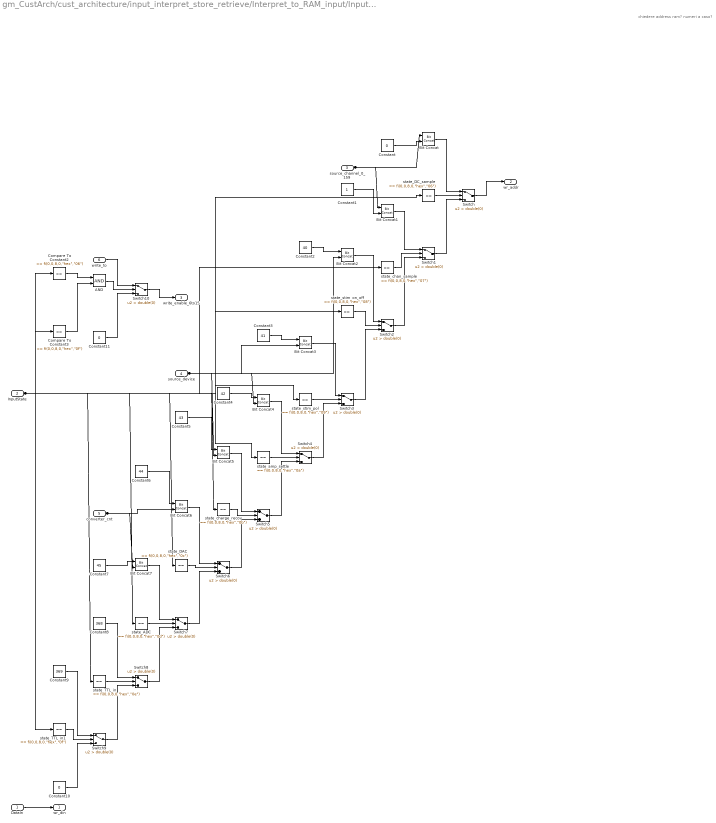
== system gm_CustArch/cust_architecture/input_interpret_store_retrieve/Interpret_to_RAM_input/Input State to RAM address (to write) ==
  note: chiedere address ram? numeri a caso?
  DataIn : Inport  OutDataTypeStr=uint16  PortDimensions=1  SampleTime=1
  InputState : Inport  Port=2  OutDataTypeStr=uint8  PortDimensions=1  SampleTime=1
  source_channel_0_159 : Inport  Port=3  OutDataTypeStr=uint8  PortDimensions=1  SampleTime=1
  source_device : Inport  Port=4  OutDataTypeStr=fixdt(0, 3, 0)  PortDimensions=1  SampleTime=1
  converter_cnt : Inport  Port=5  OutDataTypeStr=fixdt(0, 3, 0)  PortDimensions=1  SampleTime=1
  write_to : Inport  Port=6  OutDataTypeStr=boolean  PortDimensions=1  SampleTime=1
  AND : Logic  AllPortsSameDT=off  OutDataTypeStr=boolean  SampleTime=1
  Bit Concat{,1..7} (8 alike) : hdlsllib/Logic and Bit Operations/Bit Concat  numInputs=2
  Compare To Constant2 : simulink/Logic and Bit Operations/Compare To Constant  relop=>=  const="fi(0,0,8,0,\"hex\",\"06\")"  OutDataTypeStr=boolean
  Compare To Constant3 : simulink/Logic and Bit Operations/Compare To Constant  relop=<=  const="fi(0,0,8,0,\"hex\",\"0f\")"  OutDataTypeStr=boolean
  Constant : Constant  Value=0  OutDataTypeStr=boolean  SampleTime=1
  Constant1 : Constant  OutDataTypeStr=boolean  SampleTime=1
  Constant10 : Constant  Value=0  OutDataTypeStr=fixdt(0, 9, 1000)  SampleTime=1
  Constant11 : Constant  Value=0  OutDataTypeStr=boolean  SampleTime=1
  Constant2 : Constant  Value=40  OutDataTypeStr=fixdt(0, 6, 0)  SampleTime=1
  Constant3 : Constant  Value=41  OutDataTypeStr=fixdt(0, 6, 0)  SampleTime=1
  Constant4 : Constant  Value=42  OutDataTypeStr=fixdt(0, 6, 0)  SampleTime=1
  Constant5 : Constant  Value=43  OutDataTypeStr=fixdt(0, 6, 0)  SampleTime=1
  Constant6 : Constant  Value=44  OutDataTypeStr=fixdt(0, 6, 0)  SampleTime=1
  Constant7 : Constant  Value=45  OutDataTypeStr=fixdt(0, 6, 0)  SampleTime=1
  Constant8 : Constant  Value=368  OutDataTypeStr=fixdt(0, 9, 0)  SampleTime=1
  Constant9 : Constant  Value=369  OutDataTypeStr=fixdt(0, 9, 0)  SampleTime=1
  Switch{,1..9} (10 alike) : Switch  Criteria=u2 > Threshold  Threshold=double(0)  OutDataTypeStr=fixdt(0, 9, 0)  SampleTime=1
  Switch10 : Switch  Criteria=u2 > Threshold  Threshold=double(0)  OutDataTypeStr=boolean  SampleTime=1
  state_ADC : simulink/Logic and Bit Operations/Compare To Constant  relop===  const="fi(0,0,8,0,\"hex\",\"0d\")"  OutDataTypeStr=boolean
  state_DAC : simulink/Logic and Bit Operations/Compare To Constant  relop===  const="fi(0,0,8,0,\"hex\",\"0c\")"  OutDataTypeStr=boolean
  state_DC_sample : simulink/Logic and Bit Operations/Compare To Constant  relop===  const="fi(0,0,8,0,\"hex\",\"06\")"  OutDataTypeStr=boolean
  state_TTL_in : simulink/Logic and Bit Operations/Compare To Constant  relop===  const="fi(0,0,8,0,\"hex\",\"0e\")"  OutDataTypeStr=boolean
  state_TTL_in1 : simulink/Logic and Bit Operations/Compare To Constant  relop===  const="fi(0,0,8,0,\"hex\",\"0f\")"  OutDataTypeStr=boolean
  state_amp_settle : simulink/Logic and Bit Operations/Compare To Constant  relop===  const="fi(0,0,8,0,\"hex\",\"0a\")"  OutDataTypeStr=boolean
  state_chan_sample : simulink/Logic and Bit Operations/Compare To Constant  relop===  const="fi(0,0,8,0,\"hex\",\"07\")"  OutDataTypeStr=boolean
  state_charge_recov : simulink/Logic and Bit Operations/Compare To Constant  relop===  const="fi(0,0,8,0,\"hex\",\"0b\")"  OutDataTypeStr=boolean
  state_stim_on_off : simulink/Logic and Bit Operations/Compare To Constant  relop===  const="fi(0,0,8,0,\"hex\",\"08\")"  OutDataTypeStr=boolean
  state_stim_pol : simulink/Logic and Bit Operations/Compare To Constant  relop===  const="fi(0,0,8,0,\"hex\",\"09\")"  OutDataTypeStr=boolean
  wr_din : Outport  VectorParamsAs1DForOutWhenUnconnected=off
  wr_addr : Outport  Port=2  OutDataTypeStr=fixdt(0,9,0)  VectorParamsAs1DForOutWhenUnconnected=off
  write_enable_6to15 : Outport  Port=3  OutDataTypeStr=boolean  VectorParamsAs1DForOutWhenUnconnected=off
  wires:
  DataIn/1 -> wr_din/1
  InputState/1 -> state_stim_pol/1, state_stim_on_off/1, state_charge_recov/1, state_chan_sample/1, state_amp_settle/1, state_TTL_in1/1, state_TTL_in/1, state_DC_sample/1, state_DAC/1, state_ADC/1, Compare To Constant3/1, Compare To Constant2/1
  source_channel_0_159/1 -> Bit Concat1/1, Bit Concat/1
  source_device/1 -> Bit Concat5/2, Bit Concat4/2, Bit Concat3/2, Bit Concat2/2
  converter_cnt/1 -> Bit Concat7/2, Bit Concat6/2
  write_to/1 -> Switch10/1
  AND/1 -> Switch10/2
  Bit Concat/1 -> Switch/1
  Bit Concat1/1 -> Switch1/1
  Bit Concat2/1 -> Switch2/1
  Bit Concat3/1 -> Switch3/1
  Bit Concat4/1 -> Switch4/1
  Bit Concat5/1 -> Switch5/1
  Bit Concat6/1 -> Switch6/1
  Bit Concat7/1 -> Switch7/1
  Compare To Constant2/1 -> AND/1
  Compare To Constant3/1 -> AND/2
  Constant/1 -> Bit Concat/2
  Constant1/1 -> Bit Concat1/2
  Constant10/1 -> Switch9/3
  Constant11/1 -> Switch10/3
  Constant2/1 -> Bit Concat2/1
  Constant3/1 -> Bit Concat3/1
  Constant4/1 -> Bit Concat4/1
  Constant5/1 -> Bit Concat5/1
  Constant6/1 -> Bit Concat6/1
  Constant7/1 -> Bit Concat7/1
  Constant8/1 -> Switch8/1
  Constant9/1 -> Switch9/1
  Switch/1 -> wr_addr/1
  Switch1/1 -> Switch/3
  Switch10/1 -> write_enable_6to15/1
  Switch2/1 -> Switch1/3
  Switch3/1 -> Switch2/3
  Switch4/1 -> Switch3/3
  Switch5/1 -> Switch4/3
  Switch6/1 -> Switch5/3
  Switch7/1 -> Switch6/3
  Switch8/1 -> Switch7/3
  Switch9/1 -> Switch8/3
  state_ADC/1 -> Switch7/2
  state_DAC/1 -> Switch6/2
  state_DC_sample/1 -> Switch/2
  state_TTL_in/1 -> Switch8/2
  state_TTL_in1/1 -> Switch9/2
  state_amp_settle/1 -> Switch4/2
  state_chan_sample/1 -> Switch1/2
  state_charge_recov/1 -> Switch5/2
  state_stim_on_off/1 -> Switch2/2
  state_stim_pol/1 -> Switch3/2

== system gm_CustArch/cust_architecture/input_interpret_store_retrieve/Interpret_to_RAM_input/interpret data ==
  note: check ADC/DAC states
  note: count number of ADC/DAC states
  FIFO_write_to : Inport  OutDataTypeStr=boolean  PortDimensions=1  SampleTime=1
  InputState : Inport  Port=2  OutDataTypeStr=uint8  PortDimensions=1  SampleTime=1
  data_stream_enable : Inport  Port=3  OutDataTypeStr=uint8  PortDimensions=1  SampleTime=1
  Bit Slice : hdlsllib/Logic and Bit Operations/Bit Slice  lidx=double(2)  ridx=double(0)
      settings: SourceProductBaseCode=SL
  Bit Slice1 : hdlsllib/Logic and Bit Operations/Bit Slice  lidx=double(2)  ridx=double(0)
      settings: SourceProductBaseCode=SL
  HDL Counter : hdlsllib/Sources/HDL Counter  CountType=Count limited  CountInit=double(0)  CountStep=double(1)  CountMax=double(7)  CountFromType=Initial value  CountFrom=double(0)  CountResetPort=off  CountLoadPort=off  CountEnbPort=on  CountDirPort=off  CountDataType=Unsigned  CountWordLen=8  CountFracLen=0  CountSampTime=1
  "condition to count DAC or ADC " : Subsystem
  get_sources : Subsystem
  source_device : Outport  VectorParamsAs1DForOutWhenUnconnected=off
  inc_source_device : Outport  Port=2  VectorParamsAs1DForOutWhenUnconnected=off
  device_output : Outport  Port=3  VectorParamsAs1DForOutWhenUnconnected=off
  source_channel_0_159 : Outport  Port=4  VectorParamsAs1DForOutWhenUnconnected=off
  converter_cnt : Outport  Port=5  VectorParamsAs1DForOutWhenUnconnected=off
  wires:
  FIFO_write_to/1 -> "condition to count DAC or ADC "/1(fifo_write_to), get_sources/1(FIFO_write_to)
  InputState/1 -> "condition to count DAC or ADC "/2(input_state), get_sources/2(InputState)
  data_stream_enable/1 -> get_sources/3(data_stream_enable)
  Bit Slice/1 -> converter_cnt/1
  Bit Slice1/1 -> source_device/1
  HDL Counter/1 -> Bit Slice/1
  "condition to count DAC or ADC "/1(Out1) -> HDL Counter/1
  get_sources/1(source_device) -> Bit Slice1/1
  get_sources/2(dev_out_channel_0_19) -> device_output/1
  get_sources/3(source_channel) -> source_channel_0_159/1
  get_sources/4(bitmasked==0) -> inc_source_device/1

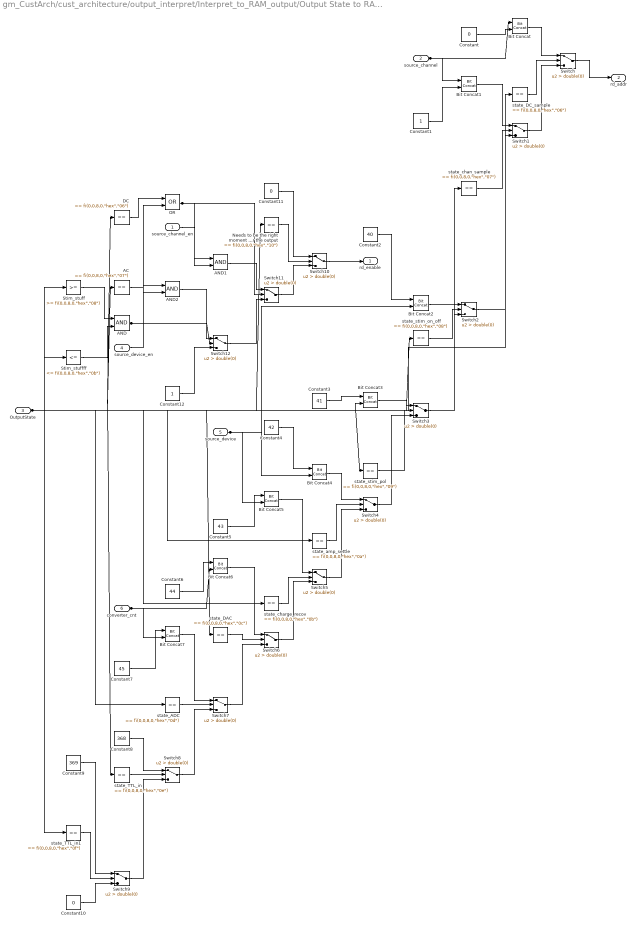
== system gm_CustArch/cust_architecture/output_interpret/Interpret_to_RAM_output/Output State to RAM address (to read) ==
  source_channel_en : Inport  OutDataTypeStr=boolean  PortDimensions=1  SampleTime=1
  source_channel : Inport  Port=2  OutDataTypeStr=uint8  PortDimensions=1  SampleTime=1
  OutputState : Inport  Port=3  OutDataTypeStr=uint8  PortDimensions=1  SampleTime=1
  source_device_en : Inport  Port=4  OutDataTypeStr=fixdt(0, 1, 0)  PortDimensions=1  SampleTime=1
  source_device : Inport  Port=5  OutDataTypeStr=fixdt(0, 3, 0)  PortDimensions=1  SampleTime=1
  converter_cnt : Inport  Port=6  OutDataTypeStr=fixdt(0, 3, 0)  PortDimensions=1  SampleTime=1
  AC : simulink/Logic and Bit Operations/Compare To Constant  relop===  const="fi(0,0,8,0,\"hex\",\"07\")"  OutDataTypeStr=boolean
  AND : Logic  AllPortsSameDT=off  OutDataTypeStr=boolean  SampleTime=1
  AND1 : Logic  AllPortsSameDT=off  OutDataTypeStr=boolean  SampleTime=1
  AND2 : Logic  AllPortsSameDT=off  OutDataTypeStr=boolean  SampleTime=1
  Bit Concat{,1..7} (8 alike) : hdlsllib/Logic and Bit Operations/Bit Concat  numInputs=2
  Constant : Constant  Value=0  OutDataTypeStr=boolean  SampleTime=1
  Constant1 : Constant  OutDataTypeStr=boolean  SampleTime=1
  Constant10 : Constant  Value=0  OutDataTypeStr=fixdt(0, 9, 1000)  SampleTime=1
  Constant11 : Constant  Value=0  OutDataTypeStr=boolean  SampleTime=1
  Constant12 : Constant  OutDataTypeStr=boolean  SampleTime=1
  Constant2 : Constant  Value=40  OutDataTypeStr=fixdt(0, 6, 0)  SampleTime=1
  Constant3 : Constant  Value=41  OutDataTypeStr=fixdt(0, 6, 0)  SampleTime=1
  Constant4 : Constant  Value=42  OutDataTypeStr=fixdt(0, 6, 0)  SampleTime=1
  Constant5 : Constant  Value=43  OutDataTypeStr=fixdt(0, 6, 0)  SampleTime=1
  Constant6 : Constant  Value=44  OutDataTypeStr=fixdt(0, 6, 0)  SampleTime=1
  Constant7 : Constant  Value=45  OutDataTypeStr=fixdt(0, 6, 0)  SampleTime=1
  Constant8 : Constant  Value=368  OutDataTypeStr=fixdt(0, 9, 0)  SampleTime=1
  Constant9 : Constant  Value=369  OutDataTypeStr=fixdt(0, 9, 0)  SampleTime=1
  DC : simulink/Logic and Bit Operations/Compare To Constant  relop===  const="fi(0,0,8,0,\"hex\",\"06\")"  OutDataTypeStr=boolean
  Needs to be the right moment for the output : simulink/Logic and Bit Operations/Compare To Constant  relop===  const="fi(0,0,8,0,\"hex\",\"10\")"  OutDataTypeStr=boolean
  OR : Logic  Operator=OR  AllPortsSameDT=off  OutDataTypeStr=boolean  SampleTime=1
  Stim_stuff : simulink/Logic and Bit Operations/Compare To Constant  relop=>=  const="fi(0,0,8,0,\"hex\",\"08\")"  OutDataTypeStr=boolean
  Stim_stuffff : simulink/Logic and Bit Operations/Compare To Constant  relop=<=  const="fi(0,0,8,0,\"hex\",\"0b\")"  OutDataTypeStr=boolean
  Switch{,1..9} (10 alike) : Switch  Criteria=u2 > Threshold  Threshold=double(0)  OutDataTypeStr=fixdt(0, 9, 0)  SampleTime=1
  Switch10 : Switch  Criteria=u2 > Threshold  Threshold=double(0)  OutDataTypeStr=boolean  SampleTime=1
  Switch11 : Switch  Criteria=u2 > Threshold  Threshold=double(0)  OutDataTypeStr=boolean  SampleTime=1
  Switch12 : Switch  Criteria=u2 > Threshold  Threshold=double(0)  OutDataTypeStr=boolean  SampleTime=1
  state_ADC : simulink/Logic and Bit Operations/Compare To Constant  relop===  const="fi(0,0,8,0,\"hex\",\"0d\")"  OutDataTypeStr=boolean
  state_DAC : simulink/Logic and Bit Operations/Compare To Constant  relop===  const="fi(0,0,8,0,\"hex\",\"0c\")"  OutDataTypeStr=boolean
  state_DC_sample : simulink/Logic and Bit Operations/Compare To Constant  relop===  const="fi(0,0,8,0,\"hex\",\"06\")"  OutDataTypeStr=boolean
  state_TTL_in : simulink/Logic and Bit Operations/Compare To Constant  relop===  const="fi(0,0,8,0,\"hex\",\"0e\")"  OutDataTypeStr=boolean
  state_TTL_in1 : simulink/Logic and Bit Operations/Compare To Constant  relop===  const="fi(0,0,8,0,\"hex\",\"0f\")"  OutDataTypeStr=boolean
  state_amp_settle : simulink/Logic and Bit Operations/Compare To Constant  relop===  const="fi(0,0,8,0,\"hex\",\"0a\")"  OutDataTypeStr=boolean
  state_chan_sample : simulink/Logic and Bit Operations/Compare To Constant  relop===  const="fi(0,0,8,0,\"hex\",\"07\")"  OutDataTypeStr=boolean
  state_charge_recov : simulink/Logic and Bit Operations/Compare To Constant  relop===  const="fi(0,0,8,0,\"hex\",\"0b\")"  OutDataTypeStr=boolean
  state_stim_on_off : simulink/Logic and Bit Operations/Compare To Constant  relop===  const="fi(0,0,8,0,\"hex\",\"08\")"  OutDataTypeStr=boolean
  state_stim_pol : simulink/Logic and Bit Operations/Compare To Constant  relop===  const="fi(0,0,8,0,\"hex\",\"09\")"  OutDataTypeStr=boolean
  rd_enable : Outport  VectorParamsAs1DForOutWhenUnconnected=off
  rd_addr : Outport  Port=2  OutDataTypeStr=fixdt(0,9,0)  VectorParamsAs1DForOutWhenUnconnected=off
  wires:
  source_channel_en/1 -> AND1/2
  source_channel/1 -> Bit Concat1/1, Bit Concat/1
  OutputState/1 -> state_stim_pol/1, state_stim_on_off/1, state_charge_recov/1, state_chan_sample/1, state_amp_settle/1, state_TTL_in1/1, state_TTL_in/1, state_DC_sample/1, state_DAC/1, state_ADC/1, Stim_stuffff/1, Stim_stuff/1, Needs to be the right moment for the output/1, DC/1, AC/1
  source_device_en/1 -> AND2/2
  source_device/1 -> Bit Concat5/2, Bit Concat4/2, Bit Concat3/2, Bit Concat2/2
  converter_cnt/1 -> Bit Concat7/2, Bit Concat6/2
  AC/1 -> OR/2
  AND/1 -> Switch12/2, AND2/1
  AND1/1 -> Switch11/1
  AND2/1 -> Switch12/1
  Bit Concat/1 -> Switch/1
  Bit Concat1/1 -> Switch1/1
  Bit Concat2/1 -> Switch2/1
  Bit Concat3/1 -> Switch3/1
  Bit Concat4/1 -> Switch4/1
  Bit Concat5/1 -> Switch5/1
  Bit Concat6/1 -> Switch6/1
  Bit Concat7/1 -> Switch7/1
  Constant/1 -> Bit Concat/2
  Constant1/1 -> Bit Concat1/2
  Constant10/1 -> Switch9/3
  Constant11/1 -> Switch10/1
  Constant12/1 -> Switch12/3
  Constant2/1 -> Bit Concat2/1
  Constant3/1 -> Bit Concat3/1
  Constant4/1 -> Bit Concat4/1
  Constant5/1 -> Bit Concat5/1
  Constant6/1 -> Bit Concat6/1
  Constant7/1 -> Bit Concat7/1
  Constant8/1 -> Switch8/1
  Constant9/1 -> Switch9/1
  DC/1 -> OR/1
  Needs to be the right moment for the output/1 -> Switch10/2
  OR/1 -> Switch11/2, AND1/1
  Stim_stuff/1 -> AND/1
  Stim_stuffff/1 -> AND/2
  Switch/1 -> rd_addr/1
  Switch1/1 -> Switch/3
  Switch10/1 -> rd_enable/1
  Switch11/1 -> Switch10/3
  Switch12/1 -> Switch11/3
  Switch2/1 -> Switch1/3
  Switch3/1 -> Switch2/3
  Switch4/1 -> Switch3/3
  Switch5/1 -> Switch4/3
  Switch6/1 -> Switch5/3
  Switch7/1 -> Switch6/3
  Switch8/1 -> Switch7/3
  Switch9/1 -> Switch8/3
  state_ADC/1 -> Switch7/2
  state_DAC/1 -> Switch6/2
  state_DC_sample/1 -> Switch/2
  state_TTL_in/1 -> Switch8/2
  state_TTL_in1/1 -> Switch9/2
  state_amp_settle/1 -> Switch4/2
  state_chan_sample/1 -> Switch1/2
  state_charge_recov/1 -> Switch5/2
  state_stim_on_off/1 -> Switch2/2
  state_stim_pol/1 -> Switch3/2

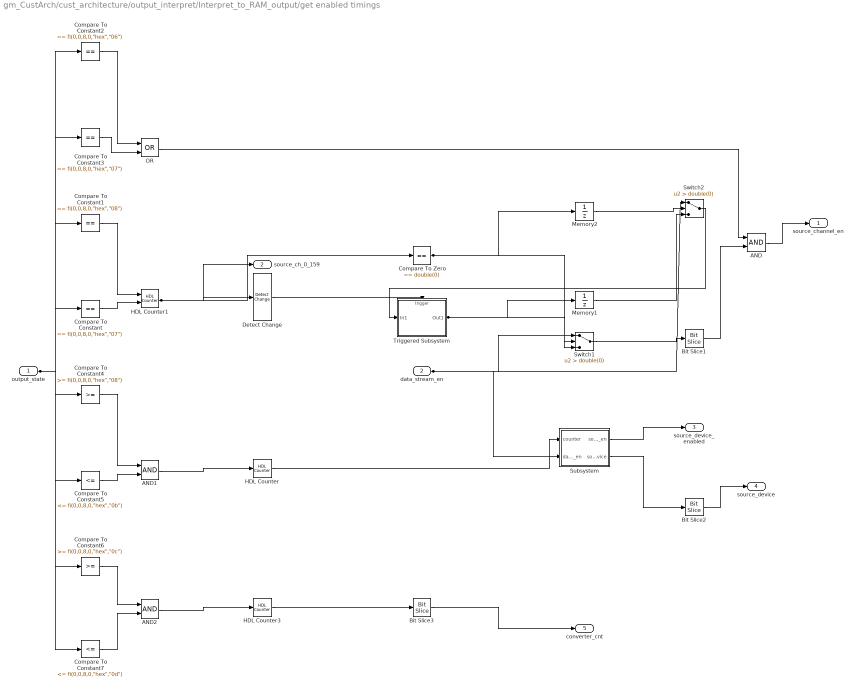
== system gm_CustArch/cust_architecture/output_interpret/Interpret_to_RAM_output/get enabled timings  ==
  output_state : Inport  OutDataTypeStr=uint8  PortDimensions=1  SampleTime=1
  data_stream_en : Inport  Port=2  OutDataTypeStr=uint8  PortDimensions=1  SampleTime=1
  AND : Logic  AllPortsSameDT=off  OutDataTypeStr=boolean  SampleTime=1
  AND1 : Logic  AllPortsSameDT=off  OutDataTypeStr=boolean  SampleTime=1
  AND2 : Logic  AllPortsSameDT=off  OutDataTypeStr=boolean  SampleTime=1
  Bit Slice1 : hdlsllib/Logic and Bit Operations/Bit Slice  lidx=double(0)  ridx=double(0)
      settings: SourceProductBaseCode=SL
  Bit Slice2 : hdlsllib/Logic and Bit Operations/Bit Slice  lidx=double(2)  ridx=double(0)
      settings: SourceProductBaseCode=SL
  Bit Slice3 : hdlsllib/Logic and Bit Operations/Bit Slice  lidx=double(2)  ridx=double(0)
      settings: SourceProductBaseCode=SL
  Compare To Constant : simulink/Logic and Bit Operations/Compare To Constant  relop===  const="fi(0,0,8,0,\"hex\",\"07\")"  OutDataTypeStr=boolean
  Compare To Constant1 : simulink/Logic and Bit Operations/Compare To Constant  relop===  const="fi(0,0,8,0,\"hex\",\"08\")"  OutDataTypeStr=boolean
  Compare To Constant2 : simulink/Logic and Bit Operations/Compare To Constant  relop===  const="fi(0,0,8,0,\"hex\",\"06\")"  OutDataTypeStr=boolean
  Compare To Constant3 : simulink/Logic and Bit Operations/Compare To Constant  relop===  const="fi(0,0,8,0,\"hex\",\"07\")"  OutDataTypeStr=boolean
  Compare To Constant4 : simulink/Logic and Bit Operations/Compare To Constant  relop=>=  const="fi(0,0,8,0,\"hex\",\"08\")"  OutDataTypeStr=boolean
  Compare To Constant5 : simulink/Logic and Bit Operations/Compare To Constant  relop=<=  const="fi(0,0,8,0,\"hex\",\"0b\")"  OutDataTypeStr=boolean
  Compare To Constant6 : simulink/Logic and Bit Operations/Compare To Constant  relop=>=  const="fi(0,0,8,0,\"hex\",\"0c\")"  OutDataTypeStr=boolean
  Compare To Constant7 : simulink/Logic and Bit Operations/Compare To Constant  relop=<=  const="fi(0,0,8,0,\"hex\",\"0d\")"  OutDataTypeStr=boolean
  Compare To Zero : simulink/Logic and Bit Operations/Compare To Constant  relop===  const=double(0)  OutDataTypeStr=boolean
  Detect Change : simulink/Logic and Bit Operations/Detect Change  vinit=0  OutDataTypeStr=boolean
  HDL Counter : hdlsllib/Sources/HDL Counter  CountType=Count limited  CountInit=double(0)  CountStep=double(1)  CountMax=double(7)  CountFromType=Initial value  CountFrom=double(0)  CountResetPort=off  CountLoadPort=off  CountEnbPort=on  CountDirPort=off  CountDataType=Unsigned  CountWordLen=8  CountFracLen=0  CountSampTime=1
  HDL Counter1 : hdlsllib/Sources/HDL Counter  CountType=Count limited  CountInit=double(0)  CountStep=double(1)  CountMax=double(159)  CountFromType=Initial value  CountFrom=double(0)  CountResetPort=on  CountLoadPort=off  CountEnbPort=on  CountDirPort=off  CountDataType=Unsigned  CountWordLen=8  CountFracLen=0  CountSampTime=1
  HDL Counter3 : hdlsllib/Sources/HDL Counter  CountType=Count limited  CountInit=double(0)  CountStep=double(1)  CountMax=double(7)  CountFromType=Initial value  CountFrom=double(0)  CountResetPort=off  CountLoadPort=off  CountEnbPort=on  CountDirPort=off  CountDataType=Unsigned  CountWordLen=8  CountFracLen=0  CountSampTime=1
  Memory1 : UnitDelay  InitialCondition=double(0)  SampleTime=1
  Memory2 : UnitDelay  InitialCondition=double(0)  SampleTime=1
  OR : Logic  Operator=OR  AllPortsSameDT=off  OutDataTypeStr=boolean  SampleTime=1
  Subsystem : Subsystem
  Switch1 : Switch  Criteria=u2 > Threshold  Threshold=double(0)  OutDataTypeStr=uint8  SampleTime=1
  Switch2 : Switch  Criteria=u2 > Threshold  Threshold=double(0)  OutDataTypeStr=uint8  SampleTime=1
  Triggered Subsystem : Subsystem
  source_channel_en : Outport  VectorParamsAs1DForOutWhenUnconnected=off
  source_ch_0_159 : Outport  Port=2  OutMin=0  OutMax=159  OutDataTypeStr=uint8  VectorParamsAs1DForOutWhenUnconnected=off  LockScale=on
  source_device_enabled : Outport  Port=3  VectorParamsAs1DForOutWhenUnconnected=off
  source_device : Outport  Port=4  VectorParamsAs1DForOutWhenUnconnected=off
  converter_cnt : Outport  Port=5  VectorParamsAs1DForOutWhenUnconnected=off
  wires:
  output_state/1 -> Compare To Constant7/1, Compare To Constant6/1, Compare To Constant5/1, Compare To Constant4/1, Compare To Constant3/1, Compare To Constant2/1, Compare To Constant1/1, Compare To Constant/1
  data_stream_en/1 -> Switch2/1, Switch1/1, Subsystem/2(data_stream_en)
  AND/1 -> source_channel_en/1
  AND1/1 -> HDL Counter/1
  AND2/1 -> HDL Counter3/1
  Bit Slice1/1 -> AND/2
  Bit Slice2/1 -> source_device/1
  Bit Slice3/1 -> converter_cnt/1
  Compare To Constant/1 -> HDL Counter1/2
  Compare To Constant1/1 -> HDL Counter1/1
  Compare To Constant2/1 -> OR/1
  Compare To Constant3/1 -> OR/2
  Compare To Constant4/1 -> AND1/1
  Compare To Constant5/1 -> AND1/2
  Compare To Constant6/1 -> AND2/1
  Compare To Constant7/1 -> AND2/2
  Compare To Zero/1 -> Switch1/2, Memory2/1
  Detect Change/1 -> Triggered Subsystem/Trigger
  HDL Counter/1 -> Subsystem/1("counter ")
  HDL Counter1/1 -> Compare To Zero/1, Detect Change/1, source_ch_0_159/1
  HDL Counter3/1 -> Bit Slice3/1
  Memory1/1 -> Switch2/3
  Memory2/1 -> Switch2/2
  OR/1 -> AND/1
  Subsystem/1(source_device_en) -> source_device_enabled/1
  Subsystem/2(source_device) -> Bit Slice2/1
  Switch1/1 -> Bit Slice1/1
  Switch2/1 -> Triggered Subsystem/1(In1)
  Triggered Subsystem/1(Out1) -> Switch1/3, Memory1/1
